simulink model "ModelE"  (R2018a)
settings: Solver=ode23  StartTime=0.0  StopTime=.1  MaxStep=1e-6  RelTol=1e-3
values from neighbouring files (symbols this model uses):
  WidthP = 60    [parameter_set.m]
libraries: powerlib x17, simulink x1
settings Model: Creator=ivank  LastModifiedBy=ivank
settings SolverCC: InitialStep=1e-8  ZeroCrossAlgorithm=Adaptive
settings DebuggingCC: MaxConsecutiveZCsMsg=none  MaskedZcDiagnostic=none  IgnoredZcDiagnostic=none

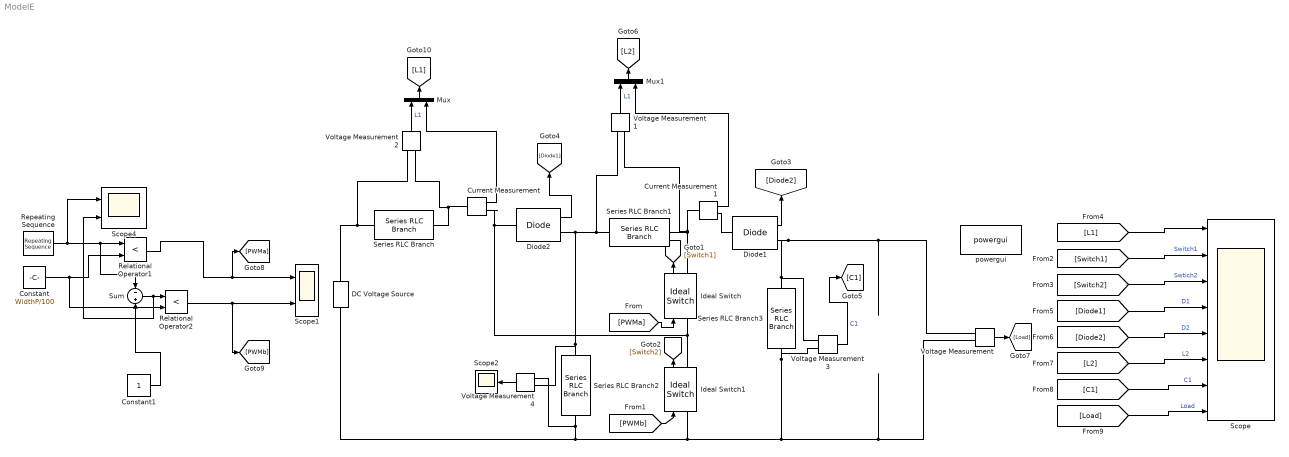
== system ModelE ==
  Constant : Constant  Value=WidthP/100
  Constant1 : Constant
  Current Measurement : powerlib/Measurements/Current Measurement  PhasorSimulation=off  OutputType=Complex  PSBequivalent=0
  Current Measurement1 : powerlib/Measurements/Current Measurement  PhasorSimulation=off  OutputType=Complex  PSBequivalent=0
  DC Voltage Source : powerlib/Electrical Sources/DC Voltage Source  Amplitude=15  Measurements=None
  Diode1 : powerlib/Power Electronics/Diode  Ron=0.001  Lon=0  Vf=0.8  IC=0  UseSnubber=0  Rs=500  Cs=250e-9  Measurements=on
  Diode2 : powerlib/Power Electronics/Diode  Ron=0.001  Lon=0  Vf=0.8  IC=0  UseSnubber=0  Rs=500  Cs=250e-9  Measurements=on
  Ideal Switch : powerlib/Power Electronics/Ideal Switch  Ron=0.00001  Lon=0  IC=0  Rs=1e9  Cs=inf  Measurements=on
  Ideal Switch1 : powerlib/Power Electronics/Ideal Switch  Ron=0.00001  Lon=0  IC=0  Rs=1e9  Cs=inf  Measurements=on
  Mux : Mux  Inputs=2
  Mux1 : Mux  Inputs=2
  Relational Operator1 : RelationalOperator  Operator=<  OutDataTypeStr=boolean  RndMeth=Simplest
  Relational Operator2 : RelationalOperator  Operator=<  OutDataTypeStr=boolean  RndMeth=Simplest
  Repeating Sequence : simulink/Sources/Repeating Sequence  rep_seq_t=[0 1/2 1]*(1/500000)  rep_seq_y=[0 1 0]
  Scope : Scope  NumInputPorts=8
  Scope1 : Scope  NumInputPorts=2
  Scope2 : Scope
  Scope4 : Scope  NumInputPorts=2
  Series RLC Branch : powerlib/Elements/Series RLC Branch  LConnTagsString=__new0  RConnTagsString=__new0  BranchType=L  Resistance=1  Inductance=(150e-6)  SetiL0=off  InitialCurrent=0  Capacitance=1e-6  Setx0=off  InitialVoltage=0  Measurements=None
  Series RLC Branch1 : powerlib/Elements/Series RLC Branch  LConnTagsString=__new0  RConnTagsString=__new0  BranchType=L  Resistance=1  Inductance=150e-6  SetiL0=off  InitialCurrent=0  Capacitance=1e-6  Setx0=off  InitialVoltage=0  Measurements=None
  Series RLC Branch2 : powerlib/Elements/Series RLC Branch  LConnTagsString=__new0  RConnTagsString=__new0  BranchType=C  Resistance=1  Inductance=1e-3  SetiL0=off  InitialCurrent=0  Capacitance=220e-6  Setx0=off  InitialVoltage=0  Measurements=None
  Series RLC Branch3 : powerlib/Elements/Series RLC Branch  LConnTagsString=__new0  RConnTagsString=__new0  BranchType=C  Resistance=1  Inductance=1e-3  SetiL0=off  InitialCurrent=0  Capacitance=220e-6  Setx0=off  InitialVoltage=0  Measurements=None
  Sum : Sum  Inputs=-+
  Voltage Measurement{,1..4} (5 alike) : powerlib/Measurements/Voltage Measurement  PhasorSimulation=off  OutputType=Complex  PSBequivalent=0
  powergui : powerlib/powergui  Priority=1  SimulationMode=Continuous  SampleTime=50e-6  frequency=60  Iterations=50  frequencyindice=0  Pbase=100e6  ErrMax=1e-4  UnitsV=kV  UnitsW=MW  buscounter=0  FunctionMessages=off  echomessages=off  EnableUseOfTLC=off  CurrentSourceSwitches=off  DisableSnubberDevices=off  DisableRonSwitches=off  DisableVfSwitches=off  DisplayEquations=off  SolverType=Tustin/Backward Euler (TBE)  Interpol=off  ExternalGateDelay=off  methode=off  Ts=100  x0status=blocks  SPID=on  SwTol=0  HookPort=off  RestoreLinks=warning  ResistiveCurrentMeasurement=off  Frange=[0:2:500]  Ylog=off  Xlog=on  ShowGrid=off  save=off  variable=ZData  structure=0  ZoomFFT=off  StartTime=0.0  cycles=1  DisplayStyle=1  fundamental=60  FreqAxis=off  MaxFrequency=1000  frequencyindicesteady=1  RmsSteady=1  display=off
  wires:
  Constant1/1 -> Sum/2
  Sum/1 -> Scope4/2, Relational Operator2/1
  Repeating Sequence/1 -> Scope4/1, Sum/1, Relational Operator1/1
  Relational Operator1/1 -> [PWMa], Scope1/1
  Relational Operator2/1 -> [PWMb], Scope1/2
  Constant/1 -> Relational Operator2/2, Relational Operator1/2
  [PWMa] -> Ideal Switch/1
  [PWMb] -> Ideal Switch1/1
  Diode2/1 -> [Diode1]
  Current Measurement/1 -> Mux/2
  Voltage Measurement2/1 -> Mux/1  "L1"
  Mux/1 -> [L1]
  Ideal Switch/1 -> [Switch1]
  Ideal Switch1/1 -> [Switch2]
  Voltage Measurement/1 -> [Load]
  Voltage Measurement3/1 -> [C1]  "C1"
  Diode1/1 -> [Diode2]
  Mux1/1 -> [L2]
  Current Measurement1/1 -> Mux1/2
  Voltage Measurement1/1 -> Mux1/1  "L1"
  [Load] -> Scope/8  "Load"
  [C1] -> Scope/7  "C1"
  [Diode2] -> Scope/5  "D2"
  [Diode1] -> Scope/4  "D1"
  [Switch1] -> Scope/2  "Switch1"
  [L1] -> Scope/1
  [Switch2] -> Scope/3  "Swtich2"
  [L2] -> Scope/6  "L2"
  Voltage Measurement4/1 -> Scope2/1
  connections:
  Series RLC Branch1/LConn1 -- Voltage Measurement1/LConn2 -- Series RLC Branch2/LConn1 -- Voltage Measurement4/LConn1 -- Diode2/RConn1
  Diode1/RConn1 -- Voltage Measurement3/LConn1 -- Series RLC Branch3/LConn1 -- Voltage Measurement/LConn1
  Series RLC Branch2/RConn1 -- Voltage Measurement4/LConn2 -- DC Voltage Source/LConn1 -- Ideal Switch1/LConn1 -- Voltage Measurement/LConn2 -- Series RLC Branch3/RConn1 -- Voltage Measurement3/LConn2
  Voltage Measurement2/LConn1 -- Series RLC Branch/RConn1 -- Current Measurement/LConn1
  Series RLC Branch/LConn1 -- Voltage Measurement2/LConn2 -- DC Voltage Source/RConn1
  Current Measurement/RConn1 -- Diode2/LConn1 -- Ideal Switch1/RConn1 -- Ideal Switch/LConn1
  Ideal Switch/RConn1 -- Voltage Measurement1/LConn1 -- Current Measurement1/LConn1 -- Series RLC Branch1/RConn1
  Diode1/LConn1 -- Current Measurement1/RConn1
